simulink model "CL_interconnection_modal_control_2_1_1"  (R2025b)
settings: Solver=VariableStepAuto  StartTime=0.0  StopTime=10.0  RelTol=1e-3
undefined symbols (not defined in the file or in its folder): alpha, Den, eta_0, Js, Num, omega, taue, xi
settings Model: Creator=flori  LastModifiedBy=flori

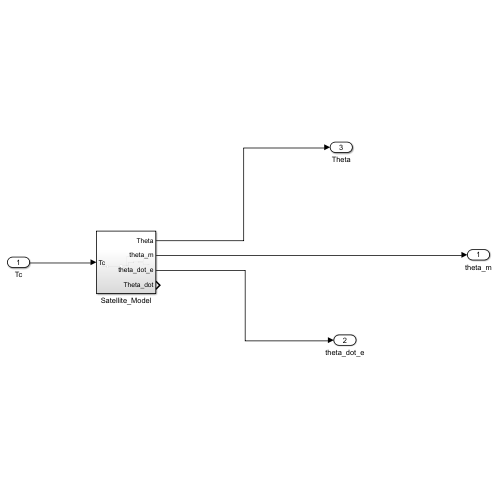
[thumbnail: Simulink's stored preview of the top-level diagram]
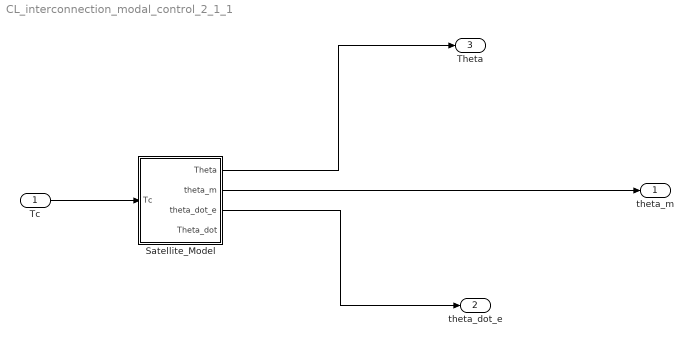
== system CL_interconnection_modal_control_2_1_1 ==
  Tc : Inport
  Satellite_Model : Subsystem
  theta_m : Outport
  theta_dot_e : Outport  Port=2
  Theta : Outport  Port=3
  wires:
  Tc/1 -> Satellite_Model/1(Tc)
  Satellite_Model/2(theta_m) -> theta_m/1
  Satellite_Model/1(Theta) -> Theta/1
  Satellite_Model/3(theta_dot_e) -> theta_dot_e/1

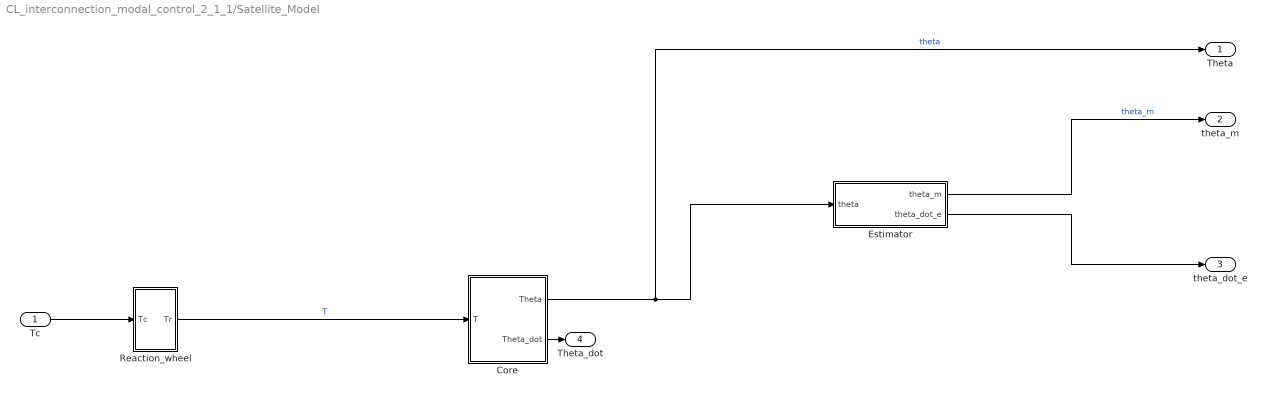
== system CL_interconnection_modal_control_2_1_1/Satellite_Model ==
  Tc : Inport
  Core : Subsystem
  Estimator : Subsystem
  Reaction_wheel : Subsystem
  Theta : Outport
  theta_m : Outport  Port=2
  theta_dot_e : Outport  Port=3
  Theta_dot : Outport  Port=4
  wires:
  Reaction_wheel/1(Tr) -> Core/1(T)  "T"
  Tc/1 -> Reaction_wheel/1(Tc)
  Core/1(Theta) -> Theta/1, Estimator/1(theta)  "theta"
  Estimator/2(theta_dot_e) -> theta_dot_e/1
  Core/2(Theta_dot) -> Theta_dot/1
  Estimator/1(theta_m) -> theta_m/1  "theta_m"

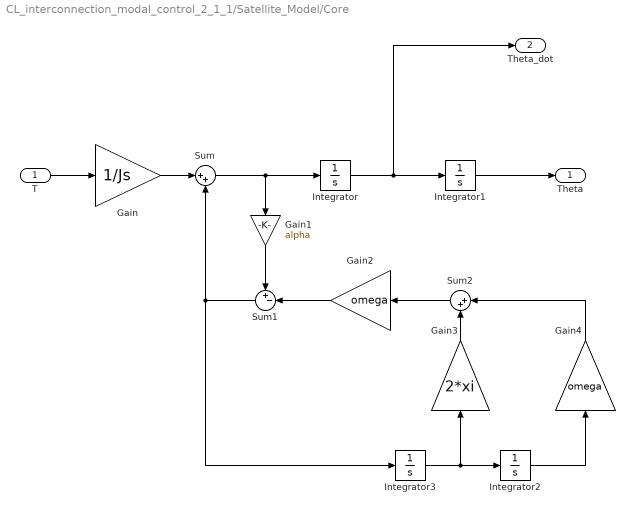
== system CL_interconnection_modal_control_2_1_1/Satellite_Model/Core ==
  T : Inport
  Gain : Gain  Gain=1/Js
  Gain1 : Gain  Gain=alpha
  Gain2 : Gain  Gain=omega
  Gain3 : Gain  Gain=2*xi
  Gain4 : Gain  Gain=omega
  Integrator : Integrator
  Integrator1 : Integrator
  Integrator2 : Integrator  InitialCondition=eta_0
  Integrator3 : Integrator
  Sum : Sum  Inputs=|++
  Sum1 : Sum  Inputs=+-|
  Sum2 : Sum  Inputs=|++
  Theta : Outport
  Theta_dot : Outport  Port=2
  wires:
  Integrator/1 -> Theta_dot/1, Integrator1/1
  Gain4/1 -> Sum2/1
  Sum/1 -> Gain1/1, Integrator/1
  Gain2/1 -> Sum1/2
  Sum1/1 -> Integrator3/1, Sum/2
  Gain1/1 -> Sum1/1
  Gain3/1 -> Sum2/2
  Integrator3/1 -> Integrator2/1, Gain3/1
  Sum2/1 -> Gain2/1
  T/1 -> Gain/1
  Integrator1/1 -> Theta/1
  Gain/1 -> Sum/1
  Integrator2/1 -> Gain4/1

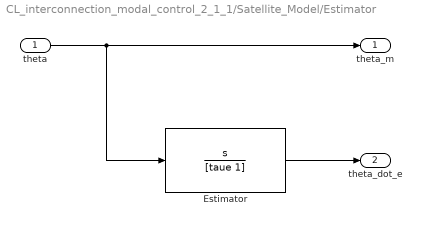
== system CL_interconnection_modal_control_2_1_1/Satellite_Model/Estimator ==
  theta : Inport
  Estimator : TransferFcn  Numerator=[1 0]  Denominator=[taue 1]
  theta_m : Outport
  theta_dot_e : Outport  Port=2
  wires:
  theta/1 -> theta_m/1, Estimator/1
  Estimator/1 -> theta_dot_e/1

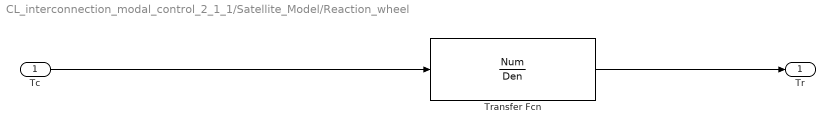
== system CL_interconnection_modal_control_2_1_1/Satellite_Model/Reaction_wheel ==
  Tc : Inport
  Transfer Fcn : TransferFcn  Numerator=Num  Denominator=Den
  Tr : Outport
  wires:
  Transfer Fcn/1 -> Tr/1
  Tc/1 -> Transfer Fcn/1
